simulink model "IEEE123bus_v2019b_Phasor_DPL_ZIPload"  (R2019b)
settings: Solver=VariableStepAuto  StartTime=0.0  StopTime=100  FixedStep=Ts  RelTol=1e-3
InitFcn:
  | a=1; % Loading Factor
  | Ts=0.1;% For Delay Blocks in Voltage Regulator Controls
  | 
  | % Simulation data for the IEEE 123 Node Test Feeder model
  | mi2km = 1.60934;%  miles to km conversion
  | ft2km = 0.0003048; % feet to km conversion
  | ms2F = 1*1e-6/(2*pi*60);% microsiemens to Farads conversion
  | 
  | %% Configuration 1
  | % Series Resitance and Reactance - ohm/mile
  | R_1 = [0.4576 0.1560 0.1535;0.1560 0.4666 0.1580;0.1535 0.1580 0.4615];
  | X_1 = [1.0780 0.5017 0.3849;0.5017 1.0482 0.4236;0.3849 0.4236 1.0651];
  | % charging susceptance - microsiemens/mile
  | B_1 = [5.6765 -1.8319 -0.6982;-1.8319 5.9809 -1.1645;-0.6982 -1.1645 5.3971];
  | 
  | R_1 = R_1/mi2km;
  | L_1 = (X_1/(2*pi*60))/mi2km;
  | C_1 =(B_1*ms2F)/mi2km;
  | 
  | %% Configuration 2 - series reactance - ohm/mile
  | R_2 = [0.4666 0.1580 0.1560;0.1580 0.4615 0.1535;0.1560 0.1535 0.4576];
  | X_2 = [1.0482 0.4236 0.5017;0.4236 1.0651 0.3849;0.5017 0.3849 1.0780];
  | % charging susceptance - microsiemens/mile
  | B_2 = [5.9809 -1.1645 -1.8319;-1.1645 5.3971 -0.6982;-1.8319 -0.6982 5.6765];
  | 
  | R_2 = R_2/mi2km;
  | L_2 = (X_2/(2*pi*60))/mi2km;
  | C_2 =(B_2*ms2F)/mi2km;
  | 
  | %% Configuration 3 - series reactance - ohm/mile
  | R_3 = [0.4615 0.1535 0.1580;0.1535 0.4576 0.1560;0.1580 0.1560 0.4666];
  | X_3 = [1.0651 0.3849 0.4236;0.3849 1.0780 0.5017;0.4236 0.5017 1.0482];
  | % charging susceptance - microsiemens/mile
  | B_3 = [5.3971 -0.6982 -1.1645;-0.6982 5.6765 -1.8319; -1.1645 -1.8319 5.9809];
  | 
  | R_3 = R_3/mi2km;
  | L_3 = (X_3/(2*pi*60))/mi2km;
  | C_3 =(B_3*ms2F)/mi2km;
  | 
  | %% Configuration 4 - series reactance - ohm/mile
  | R_4 = [0.4615 0.1580 0.1535;0.1580 0.4666 0.1560;0.1535 0.1560 0.4576];
  | X_4 = [1.0651 0.4236 0.3849;0.4236 1.0482 0.5017;0.3849 0.5017 1.0780];
  | % charging susceptance - microsiemens/mile
  | B_4 = [5.3971 -1.1645 -0.6982;-1.1645 5.9809 -1.8319;-0.6982 -1.8319 5.6765];
  | 
  | R_4 = R_4/mi2km;
  | L_4 = (X_4/(2*pi*60))/mi2km;
  | C_4 =(B_4*ms2F)/mi2km;
  | 
  | %% Configuration 5 - series reactance - ohm/mile
  | R_5 = [0.4666 0.1560 0.1580;0.1560 0.4576 0.1535;0.1580 0.1535 0.4615];
  | X_5 = [1.0482 0.5017 0.4236;0.5017 1.0780 0.3849;0.4236 0.3849 1.0651];
  | % charging susceptance - microsiemens/mile
  | B_5 = [5.9809 -1.8319 -1.1645;-1.8319 5.6765 -0.6982;-1.1645 -0.6982 5.3971];
  | 
  | R_5 = R_5/mi2km;
  | L_5 = (X_5/(2*pi*60))/mi2km;
  | C_5 =(B_5*ms2F)/mi2km;
  | 
  | %% Configuration 6 - series reactance - ohm/mile
  | ... (+68 lines)
undefined symbols (not defined in the file or in its folder): D1, Delta, find_system, j
libraries: powerlib x886, powerlib_meascontrol x31
(part 4 of 12)

== system IEEE123bus_v2019b_Phasor_DPL_ZIPload/22 Y Z ==
  Controlled Current Source : powerlib/Electrical Sources/Controlled Current Source  Initialize=off  Source_Type=AC  Amplitude=0  Phase=0  Frequency=0  Measurements=None
      settings: SourceProductName=Simscape Electrical
  Embedded MATLAB Function : MATLAB Function  TreatAsAtomicUnit=on
  Gain4 : Gain  Gain=sqrt(2)
  Gain5 : Gain  Gain=1/sqrt(2)
  Memory1 : Memory
  Rc+jXc1 : powerlib/Elements/Series RLC Branch  LConnTagsString=__new0  RConnTagsString=__new0  BranchType=R  Resistance=1e6  Inductance=1.6 / (120*pi) * 2  SetiL0=off  InitialCurrent=0  Capacitance=1e-6  Setx0=off  InitialVoltage=0  Measurements=None
      settings: SourceProductName=Simscape Electrical
  Voltage Measurement1 : powerlib/Measurements/Voltage Measurement  PhasorSimulation=on  OutputType=Complex  PSBequivalent=0
      settings: SourceProductName=Simscape Electrical
  " 2" : PMIOPort  Tag=PMCPort  Side=Left
  " 3" : PMIOPort  Tag=PMCPort  Port=2  Side=Right
  wires:
  Gain4/1 -> Memory1/1
  [v] -> Gain5/1
  Voltage Measurement1/1 -> [v]
  Gain5/1 -> Embedded MATLAB Function/1(Vmeas)
  Memory1/1 -> Controlled Current Source/1
  Embedded MATLAB Function/1(Iinj) -> Gain4/1
  connections:
  Controlled Current Source/LConn1 -- Voltage Measurement1/LConn1 -- " 2"/RConn1 -- Rc+jXc1/LConn1
  " 3"/RConn1 -- Voltage Measurement1/LConn2 -- Rc+jXc1/RConn1 -- Controlled Current Source/RConn1

== system IEEE123bus_v2019b_Phasor_DPL_ZIPload/24 ==
  2 : powerlib/Measurements/Three-Phase V-I Measurement  VoltageMeasurement=phase-to-ground  SetLabelV=on  LabelV=V24  Vpu=off  VpuLL=off  CurrentMeasurement=no  SetLabelI=on  LabelI=I800  Ipu=off  Pbase=100e6  Vbase=24900  OutputType=Complex  PhasorSimulation=on  PSBequivalent=0
      settings: SourceProductName=Simscape Electrical
  Ground82 : powerlib/Elements/Ground  LConnTagsString=a
      settings: SourceProductName=Simscape Electrical
  Ground83 : powerlib/Elements/Ground  LConnTagsString=a
      settings: SourceProductName=Simscape Electrical
  c : PMIOPort  Side=Right
  C : PMIOPort  Port=2  Side=Left
  connections:
  C/RConn1 -- 2/LConn3
  c/RConn1 -- 2/RConn3
  Ground82/LConn1 -- 2/RConn2 -- 2/RConn1
  Ground83/LConn1 -- 2/LConn2 -- 2/LConn1

== system IEEE123bus_v2019b_Phasor_DPL_ZIPload/24 Y PQ ==
  Controlled Current Source : powerlib/Electrical Sources/Controlled Current Source  Initialize=off  Source_Type=AC  Amplitude=0  Phase=0  Frequency=0  Measurements=None
      settings: SourceProductName=Simscape Electrical
  Embedded MATLAB Function : MATLAB Function  TreatAsAtomicUnit=on
  Gain4 : Gain  Gain=sqrt(2)
  Gain5 : Gain  Gain=1/sqrt(2)
  Memory1 : Memory
  Rc+jXc1 : powerlib/Elements/Series RLC Branch  LConnTagsString=__new0  RConnTagsString=__new0  BranchType=R  Resistance=1e6  Inductance=1.6 / (120*pi) * 2  SetiL0=off  InitialCurrent=0  Capacitance=1e-6  Setx0=off  InitialVoltage=0  Measurements=None
      settings: SourceProductName=Simscape Electrical
  Voltage Measurement1 : powerlib/Measurements/Voltage Measurement  PhasorSimulation=on  OutputType=Complex  PSBequivalent=0
      settings: SourceProductName=Simscape Electrical
  " 2" : PMIOPort  Tag=PMCPort  Side=Left
  " 3" : PMIOPort  Tag=PMCPort  Port=2  Side=Right
  wires:
  Embedded MATLAB Function/1(Iinj) -> Gain4/1
  Memory1/1 -> Controlled Current Source/1
  Gain5/1 -> Embedded MATLAB Function/1(Vmeas)
  Voltage Measurement1/1 -> [v]
  [v] -> Gain5/1
  Gain4/1 -> Memory1/1
  connections:
  Controlled Current Source/RConn1 -- Rc+jXc1/RConn1 -- Voltage Measurement1/LConn2 -- " 3"/RConn1
  Rc+jXc1/LConn1 -- " 2"/RConn1 -- Voltage Measurement1/LConn1 -- Controlled Current Source/LConn1

== system IEEE123bus_v2019b_Phasor_DPL_ZIPload/26 ==
  1 : powerlib/Measurements/Three-Phase V-I Measurement  VoltageMeasurement=phase-to-ground  SetLabelV=on  LabelV=V26  Vpu=off  VpuLL=off  CurrentMeasurement=no  SetLabelI=on  LabelI=I800  Ipu=off  Pbase=100e6  Vbase=24900  OutputType=Complex  PhasorSimulation=on  PSBequivalent=0
      settings: SourceProductName=Simscape Electrical
  Ground1 : powerlib/Elements/Ground  LConnTagsString=a
      settings: SourceProductName=Simscape Electrical
  Ground2 : powerlib/Elements/Ground  LConnTagsString=a
      settings: SourceProductName=Simscape Electrical
  A : PMIOPort  Side=Left
  a : PMIOPort  Port=2  Side=Right
  C : PMIOPort  Port=3  Side=Left
  c : PMIOPort  Port=4  Side=Right
  connections:
  1/LConn2 -- Ground2/LConn1
  c/RConn1 -- 1/RConn3
  1/RConn2 -- Ground1/LConn1
  C/RConn1 -- 1/LConn3
  a/RConn1 -- 1/RConn1
  A/RConn1 -- 1/LConn1

== system IEEE123bus_v2019b_Phasor_DPL_ZIPload/27 ==
  1 : powerlib/Measurements/Three-Phase V-I Measurement  VoltageMeasurement=phase-to-ground  SetLabelV=on  LabelV=V27  Vpu=off  VpuLL=off  CurrentMeasurement=no  SetLabelI=on  LabelI=I800  Ipu=off  Pbase=100e6  Vbase=24900  OutputType=Complex  PhasorSimulation=on  PSBequivalent=0
      settings: SourceProductName=Simscape Electrical
  Ground1 : powerlib/Elements/Ground  LConnTagsString=a
      settings: SourceProductName=Simscape Electrical
  Ground2 : powerlib/Elements/Ground  LConnTagsString=a
      settings: SourceProductName=Simscape Electrical
  A : PMIOPort  Side=Left
  a : PMIOPort  Port=2  Side=Right
  C : PMIOPort  Port=3  Side=Left
  c : PMIOPort  Port=4  Side=Right
  connections:
  A/RConn1 -- 1/LConn1
  a/RConn1 -- 1/RConn1
  C/RConn1 -- 1/LConn3
  1/RConn2 -- Ground1/LConn1
  c/RConn1 -- 1/RConn3
  1/LConn2 -- Ground2/LConn1

== system IEEE123bus_v2019b_Phasor_DPL_ZIPload/28 Y I ==
  Controlled Current Source : powerlib/Electrical Sources/Controlled Current Source  Initialize=off  Source_Type=AC  Amplitude=0  Phase=0  Frequency=0  Measurements=None
      settings: SourceProductName=Simscape Electrical
  Embedded MATLAB Function : MATLAB Function  TreatAsAtomicUnit=on
  Gain4 : Gain  Gain=sqrt(2)
  Gain5 : Gain  Gain=1/sqrt(2)
  Memory1 : Memory
  Rc+jXc1 : powerlib/Elements/Series RLC Branch  LConnTagsString=__new0  RConnTagsString=__new0  BranchType=R  Resistance=1e6  Inductance=1.6 / (120*pi) * 2  SetiL0=off  InitialCurrent=0  Capacitance=1e-6  Setx0=off  InitialVoltage=0  Measurements=None
      settings: SourceProductName=Simscape Electrical
  Voltage Measurement1 : powerlib/Measurements/Voltage Measurement  PhasorSimulation=on  OutputType=Complex  PSBequivalent=0
      settings: SourceProductName=Simscape Electrical
  " 2" : PMIOPort  Tag=PMCPort  Side=Left
  " 3" : PMIOPort  Tag=PMCPort  Port=2  Side=Right
  wires:
  Embedded MATLAB Function/1(Iinj) -> Gain4/1
  Memory1/1 -> Controlled Current Source/1
  Gain5/1 -> Embedded MATLAB Function/1(Vmeas)
  Voltage Measurement1/1 -> [v]
  [v] -> Gain5/1
  Gain4/1 -> Memory1/1
  connections:
  Controlled Current Source/RConn1 -- Rc+jXc1/RConn1 -- Voltage Measurement1/LConn2 -- " 3"/RConn1
  Rc+jXc1/LConn1 -- " 2"/RConn1 -- Voltage Measurement1/LConn1 -- Controlled Current Source/LConn1

== system IEEE123bus_v2019b_Phasor_DPL_ZIPload/29 Y Z ==
  Controlled Current Source : powerlib/Electrical Sources/Controlled Current Source  Initialize=off  Source_Type=AC  Amplitude=0  Phase=0  Frequency=0  Measurements=None
      settings: SourceProductName=Simscape Electrical
  Embedded MATLAB Function : MATLAB Function  TreatAsAtomicUnit=on
  Gain4 : Gain  Gain=sqrt(2)
  Gain5 : Gain  Gain=1/sqrt(2)
  Memory1 : Memory
  Rc+jXc1 : powerlib/Elements/Series RLC Branch  LConnTagsString=__new0  RConnTagsString=__new0  BranchType=R  Resistance=1e6  Inductance=1.6 / (120*pi) * 2  SetiL0=off  InitialCurrent=0  Capacitance=1e-6  Setx0=off  InitialVoltage=0  Measurements=None
      settings: SourceProductName=Simscape Electrical
  Voltage Measurement1 : powerlib/Measurements/Voltage Measurement  PhasorSimulation=on  OutputType=Complex  PSBequivalent=0
      settings: SourceProductName=Simscape Electrical
  " 2" : PMIOPort  Tag=PMCPort  Side=Left
  " 3" : PMIOPort  Tag=PMCPort  Port=2  Side=Right
  wires:
  Embedded MATLAB Function/1(Iinj) -> Gain4/1
  Memory1/1 -> Controlled Current Source/1
  Gain5/1 -> Embedded MATLAB Function/1(Vmeas)
  Voltage Measurement1/1 -> [v]
  [v] -> Gain5/1
  Gain4/1 -> Memory1/1
  connections:
  Controlled Current Source/RConn1 -- Rc+jXc1/RConn1 -- Voltage Measurement1/LConn2 -- " 3"/RConn1
  Rc+jXc1/LConn1 -- " 2"/RConn1 -- Voltage Measurement1/LConn1 -- Controlled Current Source/LConn1

== system IEEE123bus_v2019b_Phasor_DPL_ZIPload/3 ==
  2 : powerlib/Measurements/Three-Phase V-I Measurement  VoltageMeasurement=phase-to-ground  SetLabelV=on  LabelV=V3  Vpu=off  VpuLL=off  CurrentMeasurement=no  SetLabelI=on  LabelI=I800  Ipu=off  Pbase=100e6  Vbase=24900  OutputType=Complex  PhasorSimulation=on  PSBequivalent=0
      settings: SourceProductName=Simscape Electrical
  Ground82 : powerlib/Elements/Ground  LConnTagsString=a
      settings: SourceProductName=Simscape Electrical
  Ground83 : powerlib/Elements/Ground  LConnTagsString=a
      settings: SourceProductName=Simscape Electrical
  c : PMIOPort  Side=Right
  C : PMIOPort  Port=2  Side=Left
  connections:
  C/RConn1 -- 2/LConn3
  c/RConn1 -- 2/RConn3
  2/RConn2 -- 2/RConn1 -- Ground82/LConn1
  2/LConn2 -- 2/LConn1 -- Ground83/LConn1

== system IEEE123bus_v2019b_Phasor_DPL_ZIPload/30 Y PQ ==
  Controlled Current Source : powerlib/Electrical Sources/Controlled Current Source  Initialize=off  Source_Type=AC  Amplitude=0  Phase=0  Frequency=0  Measurements=None
      settings: SourceProductName=Simscape Electrical
  Embedded MATLAB Function : MATLAB Function  TreatAsAtomicUnit=on
  Gain4 : Gain  Gain=sqrt(2)
  Gain5 : Gain  Gain=1/sqrt(2)
  Memory1 : Memory
  Rc+jXc1 : powerlib/Elements/Series RLC Branch  LConnTagsString=__new0  RConnTagsString=__new0  BranchType=R  Resistance=1e6  Inductance=1.6 / (120*pi) * 2  SetiL0=off  InitialCurrent=0  Capacitance=1e-6  Setx0=off  InitialVoltage=0  Measurements=None
      settings: SourceProductName=Simscape Electrical
  Voltage Measurement1 : powerlib/Measurements/Voltage Measurement  PhasorSimulation=on  OutputType=Complex  PSBequivalent=0
      settings: SourceProductName=Simscape Electrical
  " 2" : PMIOPort  Tag=PMCPort  Side=Left
  " 3" : PMIOPort  Tag=PMCPort  Port=2  Side=Right
  wires:
  Embedded MATLAB Function/1(Iinj) -> Gain4/1
  Memory1/1 -> Controlled Current Source/1
  Gain5/1 -> Embedded MATLAB Function/1(Vmeas)
  Voltage Measurement1/1 -> [v]
  [v] -> Gain5/1
  Gain4/1 -> Memory1/1
  connections:
  Controlled Current Source/RConn1 -- Rc+jXc1/RConn1 -- Voltage Measurement1/LConn2 -- " 3"/RConn1
  Rc+jXc1/LConn1 -- " 2"/RConn1 -- Voltage Measurement1/LConn1 -- Controlled Current Source/LConn1

== system IEEE123bus_v2019b_Phasor_DPL_ZIPload/31 ==
  2 : powerlib/Measurements/Three-Phase V-I Measurement  VoltageMeasurement=phase-to-ground  SetLabelV=on  LabelV=V31  Vpu=off  VpuLL=off  CurrentMeasurement=no  SetLabelI=on  LabelI=I800  Ipu=off  Pbase=100e6  Vbase=24900  OutputType=Complex  PhasorSimulation=on  PSBequivalent=0
      settings: SourceProductName=Simscape Electrical
  Ground82 : powerlib/Elements/Ground  LConnTagsString=a
      settings: SourceProductName=Simscape Electrical
  Ground83 : powerlib/Elements/Ground  LConnTagsString=a
      settings: SourceProductName=Simscape Electrical
  c : PMIOPort  Side=Right
  C : PMIOPort  Port=2  Side=Left
  connections:
  2/LConn1 -- 2/LConn2 -- Ground83/LConn1
  2/RConn1 -- 2/RConn2 -- Ground82/LConn1
  c/RConn1 -- 2/RConn3
  C/RConn1 -- 2/LConn3

== system IEEE123bus_v2019b_Phasor_DPL_ZIPload/31 Y PQ ==
  Controlled Current Source : powerlib/Electrical Sources/Controlled Current Source  Initialize=off  Source_Type=AC  Amplitude=0  Phase=0  Frequency=0  Measurements=None
      settings: SourceProductName=Simscape Electrical
  Embedded MATLAB Function : MATLAB Function  TreatAsAtomicUnit=on
  Gain4 : Gain  Gain=sqrt(2)
  Gain5 : Gain  Gain=1/sqrt(2)
  Memory1 : Memory
  Rc+jXc1 : powerlib/Elements/Series RLC Branch  LConnTagsString=__new0  RConnTagsString=__new0  BranchType=R  Resistance=1e6  Inductance=1.6 / (120*pi) * 2  SetiL0=off  InitialCurrent=0  Capacitance=1e-6  Setx0=off  InitialVoltage=0  Measurements=None
      settings: SourceProductName=Simscape Electrical
  Voltage Measurement1 : powerlib/Measurements/Voltage Measurement  PhasorSimulation=on  OutputType=Complex  PSBequivalent=0
      settings: SourceProductName=Simscape Electrical
  " 2" : PMIOPort  Tag=PMCPort  Side=Left
  " 3" : PMIOPort  Tag=PMCPort  Port=2  Side=Right
  wires:
  Gain4/1 -> Memory1/1
  [v] -> Gain5/1
  Voltage Measurement1/1 -> [v]
  Gain5/1 -> Embedded MATLAB Function/1(Vmeas)
  Memory1/1 -> Controlled Current Source/1
  Embedded MATLAB Function/1(Iinj) -> Gain4/1
  connections:
  Controlled Current Source/LConn1 -- Voltage Measurement1/LConn1 -- " 2"/RConn1 -- Rc+jXc1/LConn1
  " 3"/RConn1 -- Voltage Measurement1/LConn2 -- Rc+jXc1/RConn1 -- Controlled Current Source/RConn1

== system IEEE123bus_v2019b_Phasor_DPL_ZIPload/32 ==
  2 : powerlib/Measurements/Three-Phase V-I Measurement  VoltageMeasurement=phase-to-ground  SetLabelV=on  LabelV=V32  Vpu=off  VpuLL=off  CurrentMeasurement=no  SetLabelI=on  LabelI=I800  Ipu=off  Pbase=100e6  Vbase=24900  OutputType=Complex  PhasorSimulation=on  PSBequivalent=0
      settings: SourceProductName=Simscape Electrical
  Ground82 : powerlib/Elements/Ground  LConnTagsString=a
      settings: SourceProductName=Simscape Electrical
  Ground83 : powerlib/Elements/Ground  LConnTagsString=a
      settings: SourceProductName=Simscape Electrical
  c : PMIOPort  Side=Right
  C : PMIOPort  Port=2  Side=Left
  connections:
  C/RConn1 -- 2/LConn3
  c/RConn1 -- 2/RConn3
  Ground82/LConn1 -- 2/RConn2 -- 2/RConn1
  Ground83/LConn1 -- 2/LConn2 -- 2/LConn1

== system IEEE123bus_v2019b_Phasor_DPL_ZIPload/32 Y PQ ==
  Controlled Current Source : powerlib/Electrical Sources/Controlled Current Source  Initialize=off  Source_Type=AC  Amplitude=0  Phase=0  Frequency=0  Measurements=None
      settings: SourceProductName=Simscape Electrical
  Embedded MATLAB Function : MATLAB Function  TreatAsAtomicUnit=on
  Gain4 : Gain  Gain=sqrt(2)
  Gain5 : Gain  Gain=1/sqrt(2)
  Memory1 : Memory
  Rc+jXc1 : powerlib/Elements/Series RLC Branch  LConnTagsString=__new0  RConnTagsString=__new0  BranchType=R  Resistance=1e6  Inductance=1.6 / (120*pi) * 2  SetiL0=off  InitialCurrent=0  Capacitance=1e-6  Setx0=off  InitialVoltage=0  Measurements=None
      settings: SourceProductName=Simscape Electrical
  Voltage Measurement1 : powerlib/Measurements/Voltage Measurement  PhasorSimulation=on  OutputType=Complex  PSBequivalent=0
      settings: SourceProductName=Simscape Electrical
  " 2" : PMIOPort  Tag=PMCPort  Side=Left
  " 3" : PMIOPort  Tag=PMCPort  Port=2  Side=Right
  wires:
  Embedded MATLAB Function/1(Iinj) -> Gain4/1
  Memory1/1 -> Controlled Current Source/1
  Gain5/1 -> Embedded MATLAB Function/1(Vmeas)
  Voltage Measurement1/1 -> [v]
  [v] -> Gain5/1
  Gain4/1 -> Memory1/1
  connections:
  Controlled Current Source/RConn1 -- Rc+jXc1/RConn1 -- Voltage Measurement1/LConn2 -- " 3"/RConn1
  Rc+jXc1/LConn1 -- " 2"/RConn1 -- Voltage Measurement1/LConn1 -- Controlled Current Source/LConn1

== system IEEE123bus_v2019b_Phasor_DPL_ZIPload/33 ==
  2 : powerlib/Measurements/Three-Phase V-I Measurement  VoltageMeasurement=phase-to-ground  SetLabelV=on  LabelV=V33  Vpu=off  VpuLL=off  CurrentMeasurement=no  SetLabelI=on  LabelI=I800  Ipu=off  Pbase=100e6  Vbase=24900  OutputType=Complex  PhasorSimulation=on  PSBequivalent=0
      settings: SourceProductName=Simscape Electrical
  Ground82 : powerlib/Elements/Ground  LConnTagsString=a
      settings: SourceProductName=Simscape Electrical
  Ground83 : powerlib/Elements/Ground  LConnTagsString=a
      settings: SourceProductName=Simscape Electrical
  a : PMIOPort  Side=Right
  A : PMIOPort  Port=2  Side=Left
  connections:
  A/RConn1 -- 2/LConn1
  a/RConn1 -- 2/RConn1
  Ground83/LConn1 -- 2/LConn2 -- 2/LConn3
  Ground82/LConn1 -- 2/RConn2 -- 2/RConn3

== system IEEE123bus_v2019b_Phasor_DPL_ZIPload/33 Y I ==
  Controlled Current Source : powerlib/Electrical Sources/Controlled Current Source  Initialize=off  Source_Type=AC  Amplitude=0  Phase=0  Frequency=0  Measurements=None
      settings: SourceProductName=Simscape Electrical
  Embedded MATLAB Function : MATLAB Function  TreatAsAtomicUnit=on
  Gain4 : Gain  Gain=sqrt(2)
  Gain5 : Gain  Gain=1/sqrt(2)
  Memory1 : Memory
  Rc+jXc1 : powerlib/Elements/Series RLC Branch  LConnTagsString=__new0  RConnTagsString=__new0  BranchType=R  Resistance=1e6  Inductance=1.6 / (120*pi) * 2  SetiL0=off  InitialCurrent=0  Capacitance=1e-6  Setx0=off  InitialVoltage=0  Measurements=None
      settings: SourceProductName=Simscape Electrical
  Voltage Measurement1 : powerlib/Measurements/Voltage Measurement  PhasorSimulation=on  OutputType=Complex  PSBequivalent=0
      settings: SourceProductName=Simscape Electrical
  " 2" : PMIOPort  Tag=PMCPort  Side=Left
  " 3" : PMIOPort  Tag=PMCPort  Port=2  Side=Right
  wires:
  Embedded MATLAB Function/1(Iinj) -> Gain4/1
  Memory1/1 -> Controlled Current Source/1
  Gain5/1 -> Embedded MATLAB Function/1(Vmeas)
  Voltage Measurement1/1 -> [v]
  [v] -> Gain5/1
  Gain4/1 -> Memory1/1
  connections:
  Controlled Current Source/RConn1 -- Rc+jXc1/RConn1 -- Voltage Measurement1/LConn2 -- " 3"/RConn1
  Rc+jXc1/LConn1 -- " 2"/RConn1 -- Voltage Measurement1/LConn1 -- Controlled Current Source/LConn1

== system IEEE123bus_v2019b_Phasor_DPL_ZIPload/34 ==
  2 : powerlib/Measurements/Three-Phase V-I Measurement  VoltageMeasurement=phase-to-ground  SetLabelV=on  LabelV=V34  Vpu=off  VpuLL=off  CurrentMeasurement=no  SetLabelI=on  LabelI=I800  Ipu=off  Pbase=100e6  Vbase=24900  OutputType=Complex  PhasorSimulation=on  PSBequivalent=0
      settings: SourceProductName=Simscape Electrical
  Ground82 : powerlib/Elements/Ground  LConnTagsString=a
      settings: SourceProductName=Simscape Electrical
  Ground83 : powerlib/Elements/Ground  LConnTagsString=a
      settings: SourceProductName=Simscape Electrical
  c : PMIOPort  Side=Right
  C : PMIOPort  Port=2  Side=Left
  connections:
  C/RConn1 -- 2/LConn3
  c/RConn1 -- 2/RConn3
  2/RConn2 -- 2/RConn1 -- Ground82/LConn1
  2/LConn2 -- 2/LConn1 -- Ground83/LConn1

== system IEEE123bus_v2019b_Phasor_DPL_ZIPload/34 Y Z ==
  Controlled Current Source : powerlib/Electrical Sources/Controlled Current Source  Initialize=off  Source_Type=AC  Amplitude=0  Phase=0  Frequency=0  Measurements=None
      settings: SourceProductName=Simscape Electrical
  Embedded MATLAB Function : MATLAB Function  TreatAsAtomicUnit=on
  Gain4 : Gain  Gain=sqrt(2)
  Gain5 : Gain  Gain=1/sqrt(2)
  Memory1 : Memory
  Rc+jXc1 : powerlib/Elements/Series RLC Branch  LConnTagsString=__new0  RConnTagsString=__new0  BranchType=R  Resistance=1e6  Inductance=1.6 / (120*pi) * 2  SetiL0=off  InitialCurrent=0  Capacitance=1e-6  Setx0=off  InitialVoltage=0  Measurements=None
      settings: SourceProductName=Simscape Electrical
  Voltage Measurement1 : powerlib/Measurements/Voltage Measurement  PhasorSimulation=on  OutputType=Complex  PSBequivalent=0
      settings: SourceProductName=Simscape Electrical
  " 2" : PMIOPort  Tag=PMCPort  Side=Left
  " 3" : PMIOPort  Tag=PMCPort  Port=2  Side=Right
  wires:
  Embedded MATLAB Function/1(Iinj) -> Gain4/1
  Memory1/1 -> Controlled Current Source/1
  Gain5/1 -> Embedded MATLAB Function/1(Vmeas)
  Voltage Measurement1/1 -> [v]
  [v] -> Gain5/1
  Gain4/1 -> Memory1/1
  connections:
  Controlled Current Source/RConn1 -- Rc+jXc1/RConn1 -- Voltage Measurement1/LConn2 -- " 3"/RConn1
  Rc+jXc1/LConn1 -- " 2"/RConn1 -- Voltage Measurement1/LConn1 -- Controlled Current Source/LConn1

== system IEEE123bus_v2019b_Phasor_DPL_ZIPload/35 D PQ ==
  Controlled Current Source : powerlib/Electrical Sources/Controlled Current Source  Initialize=off  Source_Type=AC  Amplitude=0  Phase=0  Frequency=0  Measurements=None
      settings: SourceProductName=Simscape Electrical
  Embedded MATLAB Function : MATLAB Function  TreatAsAtomicUnit=on
  Gain4 : Gain  Gain=sqrt(2)
  Gain5 : Gain  Gain=1/sqrt(2)
  Memory1 : Memory
  Rc+jXc1 : powerlib/Elements/Series RLC Branch  LConnTagsString=__new0  RConnTagsString=__new0  BranchType=R  Resistance=1e6  Inductance=1.6 / (120*pi) * 2  SetiL0=off  InitialCurrent=0  Capacitance=1e-6  Setx0=off  InitialVoltage=0  Measurements=None
      settings: SourceProductName=Simscape Electrical
  Voltage Measurement1 : powerlib/Measurements/Voltage Measurement  PhasorSimulation=on  OutputType=Complex  PSBequivalent=0
      settings: SourceProductName=Simscape Electrical
  " 2" : PMIOPort  Tag=PMCPort  Side=Left
  " 3" : PMIOPort  Tag=PMCPort  Port=2  Side=Right
  wires:
  Embedded MATLAB Function/1(Iinj) -> Gain4/1
  Memory1/1 -> Controlled Current Source/1
  Gain5/1 -> Embedded MATLAB Function/1(Vmeas)
  Voltage Measurement1/1 -> [v]
  [v] -> Gain5/1
  Gain4/1 -> Memory1/1
  connections:
  Controlled Current Source/RConn1 -- Rc+jXc1/RConn1 -- Voltage Measurement1/LConn2 -- " 3"/RConn1
  Rc+jXc1/LConn1 -- " 2"/RConn1 -- Voltage Measurement1/LConn1 -- Controlled Current Source/LConn1

== system IEEE123bus_v2019b_Phasor_DPL_ZIPload/36 ==
  1 : powerlib/Measurements/Three-Phase V-I Measurement  VoltageMeasurement=phase-to-ground  SetLabelV=on  LabelV=V36  Vpu=off  VpuLL=off  CurrentMeasurement=no  SetLabelI=on  LabelI=I800  Ipu=off  Pbase=100e6  Vbase=24900  OutputType=Complex  PhasorSimulation=on  PSBequivalent=0
      settings: SourceProductName=Simscape Electrical
  Ground1 : powerlib/Elements/Ground  LConnTagsString=a
      settings: SourceProductName=Simscape Electrical
  Ground2 : powerlib/Elements/Ground  LConnTagsString=a
      settings: SourceProductName=Simscape Electrical
  A : PMIOPort  Side=Left
  a : PMIOPort  Port=2  Side=Right
  B : PMIOPort  Port=3  Side=Left
  b : PMIOPort  Port=4  Side=Right
  connections:
  A/RConn1 -- 1/LConn1
  a/RConn1 -- 1/RConn1
  b/RConn1 -- 1/RConn2
  1/RConn3 -- Ground1/LConn1
  B/RConn1 -- 1/LConn2
  1/LConn3 -- Ground2/LConn1

== system IEEE123bus_v2019b_Phasor_DPL_ZIPload/37 ==
  2 : powerlib/Measurements/Three-Phase V-I Measurement  VoltageMeasurement=phase-to-ground  SetLabelV=on  LabelV=V37  Vpu=off  VpuLL=off  CurrentMeasurement=no  SetLabelI=on  LabelI=I800  Ipu=off  Pbase=100e6  Vbase=24900  OutputType=Complex  PhasorSimulation=on  PSBequivalent=0
      settings: SourceProductName=Simscape Electrical
  Ground82 : powerlib/Elements/Ground  LConnTagsString=a
      settings: SourceProductName=Simscape Electrical
  Ground83 : powerlib/Elements/Ground  LConnTagsString=a
      settings: SourceProductName=Simscape Electrical
  a : PMIOPort  Side=Right
  A : PMIOPort  Port=2  Side=Left
  connections:
  2/RConn3 -- 2/RConn2 -- Ground82/LConn1
  2/LConn3 -- 2/LConn2 -- Ground83/LConn1
  a/RConn1 -- 2/RConn1
  A/RConn1 -- 2/LConn1

== system IEEE123bus_v2019b_Phasor_DPL_ZIPload/37 Y Z ==
  Controlled Current Source : powerlib/Electrical Sources/Controlled Current Source  Initialize=off  Source_Type=AC  Amplitude=0  Phase=0  Frequency=0  Measurements=None
      settings: SourceProductName=Simscape Electrical
  Embedded MATLAB Function : MATLAB Function  TreatAsAtomicUnit=on
  Gain4 : Gain  Gain=sqrt(2)
  Gain5 : Gain  Gain=1/sqrt(2)
  Memory1 : Memory
  Rc+jXc1 : powerlib/Elements/Series RLC Branch  LConnTagsString=__new0  RConnTagsString=__new0  BranchType=R  Resistance=1e6  Inductance=1.6 / (120*pi) * 2  SetiL0=off  InitialCurrent=0  Capacitance=1e-6  Setx0=off  InitialVoltage=0  Measurements=None
      settings: SourceProductName=Simscape Electrical
  Voltage Measurement1 : powerlib/Measurements/Voltage Measurement  PhasorSimulation=on  OutputType=Complex  PSBequivalent=0
      settings: SourceProductName=Simscape Electrical
  " 2" : PMIOPort  Tag=PMCPort  Side=Left
  " 3" : PMIOPort  Tag=PMCPort  Port=2  Side=Right
  wires:
  Embedded MATLAB Function/1(Iinj) -> Gain4/1
  Memory1/1 -> Controlled Current Source/1
  Gain5/1 -> Embedded MATLAB Function/1(Vmeas)
  Voltage Measurement1/1 -> [v]
  [v] -> Gain5/1
  Gain4/1 -> Memory1/1
  connections:
  Controlled Current Source/RConn1 -- Rc+jXc1/RConn1 -- Voltage Measurement1/LConn2 -- " 3"/RConn1
  Rc+jXc1/LConn1 -- " 2"/RConn1 -- Voltage Measurement1/LConn1 -- Controlled Current Source/LConn1

== system IEEE123bus_v2019b_Phasor_DPL_ZIPload/38 ==
  2 : powerlib/Measurements/Three-Phase V-I Measurement  VoltageMeasurement=phase-to-ground  SetLabelV=on  LabelV=V38  Vpu=off  VpuLL=off  CurrentMeasurement=no  SetLabelI=on  LabelI=I800  Ipu=off  Pbase=100e6  Vbase=24900  OutputType=Complex  PhasorSimulation=on  PSBequivalent=0
      settings: SourceProductName=Simscape Electrical
  Ground82 : powerlib/Elements/Ground  LConnTagsString=a
      settings: SourceProductName=Simscape Electrical
  Ground83 : powerlib/Elements/Ground  LConnTagsString=a
      settings: SourceProductName=Simscape Electrical
  b : PMIOPort  Side=Right
  B : PMIOPort  Port=2  Side=Left
  connections:
  Ground82/LConn1 -- 2/RConn3 -- 2/RConn1
  Ground83/LConn1 -- 2/LConn3 -- 2/LConn1
  2/RConn2 -- b/RConn1
  2/LConn2 -- B/RConn1

== system IEEE123bus_v2019b_Phasor_DPL_ZIPload/38 Y I ==
  Controlled Current Source : powerlib/Electrical Sources/Controlled Current Source  Initialize=off  Source_Type=AC  Amplitude=0  Phase=0  Frequency=0  Measurements=None
      settings: SourceProductName=Simscape Electrical
  Embedded MATLAB Function : MATLAB Function  TreatAsAtomicUnit=on
  Gain4 : Gain  Gain=sqrt(2)
  Gain5 : Gain  Gain=1/sqrt(2)
  Memory1 : Memory
  Rc+jXc1 : powerlib/Elements/Series RLC Branch  LConnTagsString=__new0  RConnTagsString=__new0  BranchType=R  Resistance=1e6  Inductance=1.6 / (120*pi) * 2  SetiL0=off  InitialCurrent=0  Capacitance=1e-6  Setx0=off  InitialVoltage=0  Measurements=None
      settings: SourceProductName=Simscape Electrical
  Voltage Measurement1 : powerlib/Measurements/Voltage Measurement  PhasorSimulation=on  OutputType=Complex  PSBequivalent=0
      settings: SourceProductName=Simscape Electrical
  " 2" : PMIOPort  Tag=PMCPort  Side=Left
  " 3" : PMIOPort  Tag=PMCPort  Port=2  Side=Right
  wires:
  Gain4/1 -> Memory1/1
  [v] -> Gain5/1
  Voltage Measurement1/1 -> [v]
  Gain5/1 -> Embedded MATLAB Function/1(Vmeas)
  Memory1/1 -> Controlled Current Source/1
  Embedded MATLAB Function/1(Iinj) -> Gain4/1
  connections:
  Controlled Current Source/LConn1 -- Voltage Measurement1/LConn1 -- " 2"/RConn1 -- Rc+jXc1/LConn1
  " 3"/RConn1 -- Voltage Measurement1/LConn2 -- Rc+jXc1/RConn1 -- Controlled Current Source/RConn1

== system IEEE123bus_v2019b_Phasor_DPL_ZIPload/39 ==
  2 : powerlib/Measurements/Three-Phase V-I Measurement  VoltageMeasurement=phase-to-ground  SetLabelV=on  LabelV=V39  Vpu=off  VpuLL=off  CurrentMeasurement=no  SetLabelI=on  LabelI=I800  Ipu=off  Pbase=100e6  Vbase=24900  OutputType=Complex  PhasorSimulation=on  PSBequivalent=0
      settings: SourceProductName=Simscape Electrical
  Ground82 : powerlib/Elements/Ground  LConnTagsString=a
      settings: SourceProductName=Simscape Electrical
  Ground83 : powerlib/Elements/Ground  LConnTagsString=a
      settings: SourceProductName=Simscape Electrical
  b : PMIOPort  Side=Right
  B : PMIOPort  Port=2  Side=Left
  connections:
  2/LConn2 -- B/RConn1
  2/RConn2 -- b/RConn1
  2/LConn1 -- 2/LConn3 -- Ground83/LConn1
  2/RConn1 -- 2/RConn3 -- Ground82/LConn1

== system IEEE123bus_v2019b_Phasor_DPL_ZIPload/39 Y PQ ==
  Controlled Current Source : powerlib/Electrical Sources/Controlled Current Source  Initialize=off  Source_Type=AC  Amplitude=0  Phase=0  Frequency=0  Measurements=None
      settings: SourceProductName=Simscape Electrical
  Embedded MATLAB Function : MATLAB Function  TreatAsAtomicUnit=on
  Gain4 : Gain  Gain=sqrt(2)
  Gain5 : Gain  Gain=1/sqrt(2)
  Memory1 : Memory
  Rc+jXc1 : powerlib/Elements/Series RLC Branch  LConnTagsString=__new0  RConnTagsString=__new0  BranchType=R  Resistance=1e6  Inductance=1.6 / (120*pi) * 2  SetiL0=off  InitialCurrent=0  Capacitance=1e-6  Setx0=off  InitialVoltage=0  Measurements=None
      settings: SourceProductName=Simscape Electrical
  Voltage Measurement1 : powerlib/Measurements/Voltage Measurement  PhasorSimulation=on  OutputType=Complex  PSBequivalent=0
      settings: SourceProductName=Simscape Electrical
  " 2" : PMIOPort  Tag=PMCPort  Side=Left
  " 3" : PMIOPort  Tag=PMCPort  Port=2  Side=Right
  wires:
  Gain4/1 -> Memory1/1
  [v] -> Gain5/1
  Voltage Measurement1/1 -> [v]
  Gain5/1 -> Embedded MATLAB Function/1(Vmeas)
  Memory1/1 -> Controlled Current Source/1
  Embedded MATLAB Function/1(Iinj) -> Gain4/1
  connections:
  Controlled Current Source/LConn1 -- Voltage Measurement1/LConn1 -- " 2"/RConn1 -- Rc+jXc1/LConn1
  " 3"/RConn1 -- Voltage Measurement1/LConn2 -- Rc+jXc1/RConn1 -- Controlled Current Source/RConn1

== system IEEE123bus_v2019b_Phasor_DPL_ZIPload/4 ==
  2 : powerlib/Measurements/Three-Phase V-I Measurement  VoltageMeasurement=phase-to-ground  SetLabelV=on  LabelV=V4  Vpu=off  VpuLL=off  CurrentMeasurement=no  SetLabelI=on  LabelI=I4  Ipu=off  Pbase=100e6  Vbase=24900  OutputType=Complex  PhasorSimulation=on  PSBequivalent=0
      settings: SourceProductName=Simscape Electrical
  Ground82 : powerlib/Elements/Ground  LConnTagsString=a
      settings: SourceProductName=Simscape Electrical
  Ground83 : powerlib/Elements/Ground  LConnTagsString=a
      settings: SourceProductName=Simscape Electrical
  c : PMIOPort  Side=Right
  C : PMIOPort  Port=2  Side=Left
  connections:
  Ground83/LConn1 -- 2/LConn1 -- 2/LConn2
  Ground82/LConn1 -- 2/RConn1 -- 2/RConn2
  c/RConn1 -- 2/RConn3
  C/RConn1 -- 2/LConn3

== system IEEE123bus_v2019b_Phasor_DPL_ZIPload/41 ==
  2 : powerlib/Measurements/Three-Phase V-I Measurement  VoltageMeasurement=phase-to-ground  SetLabelV=on  LabelV=V41  Vpu=off  VpuLL=off  CurrentMeasurement=no  SetLabelI=on  LabelI=I800  Ipu=off  Pbase=100e6  Vbase=24900  OutputType=Complex  PhasorSimulation=on  PSBequivalent=0
      settings: SourceProductName=Simscape Electrical
  Ground82 : powerlib/Elements/Ground  LConnTagsString=a
      settings: SourceProductName=Simscape Electrical
  Ground83 : powerlib/Elements/Ground  LConnTagsString=a
      settings: SourceProductName=Simscape Electrical
  c : PMIOPort  Side=Right
  C : PMIOPort  Port=2  Side=Left
  connections:
  2/LConn1 -- 2/LConn2 -- Ground83/LConn1
  2/RConn1 -- 2/RConn2 -- Ground82/LConn1
  c/RConn1 -- 2/RConn3
  C/RConn1 -- 2/LConn3

== system IEEE123bus_v2019b_Phasor_DPL_ZIPload/41 Y PQ ==
  Controlled Current Source : powerlib/Electrical Sources/Controlled Current Source  Initialize=off  Source_Type=AC  Amplitude=0  Phase=0  Frequency=0  Measurements=None
      settings: SourceProductName=Simscape Electrical
  Embedded MATLAB Function : MATLAB Function  TreatAsAtomicUnit=on
  Gain4 : Gain  Gain=sqrt(2)
  Gain5 : Gain  Gain=1/sqrt(2)
  Memory1 : Memory
  Rc+jXc1 : powerlib/Elements/Series RLC Branch  LConnTagsString=__new0  RConnTagsString=__new0  BranchType=R  Resistance=1e6  Inductance=1.6 / (120*pi) * 2  SetiL0=off  InitialCurrent=0  Capacitance=1e-6  Setx0=off  InitialVoltage=0  Measurements=None
      settings: SourceProductName=Simscape Electrical
  Voltage Measurement1 : powerlib/Measurements/Voltage Measurement  PhasorSimulation=on  OutputType=Complex  PSBequivalent=0
      settings: SourceProductName=Simscape Electrical
  " 2" : PMIOPort  Tag=PMCPort  Side=Left
  " 3" : PMIOPort  Tag=PMCPort  Port=2  Side=Right
  wires:
  Gain4/1 -> Memory1/1
  [v] -> Gain5/1
  Voltage Measurement1/1 -> [v]
  Gain5/1 -> Embedded MATLAB Function/1(Vmeas)
  Memory1/1 -> Controlled Current Source/1
  Embedded MATLAB Function/1(Iinj) -> Gain4/1
  connections:
  Controlled Current Source/LConn1 -- Voltage Measurement1/LConn1 -- " 2"/RConn1 -- Rc+jXc1/LConn1
  " 3"/RConn1 -- Voltage Measurement1/LConn2 -- Rc+jXc1/RConn1 -- Controlled Current Source/RConn1

== system IEEE123bus_v2019b_Phasor_DPL_ZIPload/42 Y PQ ==
  Controlled Current Source : powerlib/Electrical Sources/Controlled Current Source  Initialize=off  Source_Type=AC  Amplitude=0  Phase=0  Frequency=0  Measurements=None
      settings: SourceProductName=Simscape Electrical
  Embedded MATLAB Function : MATLAB Function  TreatAsAtomicUnit=on
  Gain4 : Gain  Gain=sqrt(2)
  Gain5 : Gain  Gain=1/sqrt(2)
  Memory1 : Memory
  Rc+jXc1 : powerlib/Elements/Series RLC Branch  LConnTagsString=__new0  RConnTagsString=__new0  BranchType=R  Resistance=1e6  Inductance=1.6 / (120*pi) * 2  SetiL0=off  InitialCurrent=0  Capacitance=1e-6  Setx0=off  InitialVoltage=0  Measurements=None
      settings: SourceProductName=Simscape Electrical
  Voltage Measurement1 : powerlib/Measurements/Voltage Measurement  PhasorSimulation=on  OutputType=Complex  PSBequivalent=0
      settings: SourceProductName=Simscape Electrical
  " 2" : PMIOPort  Tag=PMCPort  Side=Left
  " 3" : PMIOPort  Tag=PMCPort  Port=2  Side=Right
  wires:
  Embedded MATLAB Function/1(Iinj) -> Gain4/1
  Memory1/1 -> Controlled Current Source/1
  Gain5/1 -> Embedded MATLAB Function/1(Vmeas)
  Voltage Measurement1/1 -> [v]
  [v] -> Gain5/1
  Gain4/1 -> Memory1/1
  connections:
  Controlled Current Source/RConn1 -- Rc+jXc1/RConn1 -- Voltage Measurement1/LConn2 -- " 3"/RConn1
  Rc+jXc1/LConn1 -- " 2"/RConn1 -- Voltage Measurement1/LConn1 -- Controlled Current Source/LConn1

== system IEEE123bus_v2019b_Phasor_DPL_ZIPload/43 ==
  2 : powerlib/Measurements/Three-Phase V-I Measurement  VoltageMeasurement=phase-to-ground  SetLabelV=on  LabelV=V43  Vpu=off  VpuLL=off  CurrentMeasurement=no  SetLabelI=on  LabelI=I800  Ipu=off  Pbase=100e6  Vbase=24900  OutputType=Complex  PhasorSimulation=on  PSBequivalent=0
      settings: SourceProductName=Simscape Electrical
  Ground82 : powerlib/Elements/Ground  LConnTagsString=a
      settings: SourceProductName=Simscape Electrical
  Ground83 : powerlib/Elements/Ground  LConnTagsString=a
      settings: SourceProductName=Simscape Electrical
  b : PMIOPort  Side=Right
  B : PMIOPort  Port=2  Side=Left
  connections:
  2/LConn2 -- B/RConn1
  2/RConn2 -- b/RConn1
  2/LConn1 -- 2/LConn3 -- Ground83/LConn1
  2/RConn1 -- 2/RConn3 -- Ground82/LConn1

== system IEEE123bus_v2019b_Phasor_DPL_ZIPload/43 Y Z ==
  Controlled Current Source : powerlib/Electrical Sources/Controlled Current Source  Initialize=off  Source_Type=AC  Amplitude=0  Phase=0  Frequency=0  Measurements=None
      settings: SourceProductName=Simscape Electrical
  Embedded MATLAB Function : MATLAB Function  TreatAsAtomicUnit=on
  Gain4 : Gain  Gain=sqrt(2)
  Gain5 : Gain  Gain=1/sqrt(2)
  Memory1 : Memory
  Rc+jXc1 : powerlib/Elements/Series RLC Branch  LConnTagsString=__new0  RConnTagsString=__new0  BranchType=R  Resistance=1e6  Inductance=1.6 / (120*pi) * 2  SetiL0=off  InitialCurrent=0  Capacitance=1e-6  Setx0=off  InitialVoltage=0  Measurements=None
      settings: SourceProductName=Simscape Electrical
  Voltage Measurement1 : powerlib/Measurements/Voltage Measurement  PhasorSimulation=on  OutputType=Complex  PSBequivalent=0
      settings: SourceProductName=Simscape Electrical
  " 2" : PMIOPort  Tag=PMCPort  Side=Left
  " 3" : PMIOPort  Tag=PMCPort  Port=2  Side=Right
  wires:
  Embedded MATLAB Function/1(Iinj) -> Gain4/1
  Memory1/1 -> Controlled Current Source/1
  Gain5/1 -> Embedded MATLAB Function/1(Vmeas)
  Voltage Measurement1/1 -> [v]
  [v] -> Gain5/1
  Gain4/1 -> Memory1/1
  connections:
  Controlled Current Source/RConn1 -- Rc+jXc1/RConn1 -- Voltage Measurement1/LConn2 -- " 3"/RConn1
  Rc+jXc1/LConn1 -- " 2"/RConn1 -- Voltage Measurement1/LConn1 -- Controlled Current Source/LConn1

== system IEEE123bus_v2019b_Phasor_DPL_ZIPload/45 ==
  2 : powerlib/Measurements/Three-Phase V-I Measurement  VoltageMeasurement=phase-to-ground  SetLabelV=on  LabelV=V45  Vpu=off  VpuLL=off  CurrentMeasurement=no  SetLabelI=on  LabelI=I800  Ipu=off  Pbase=100e6  Vbase=24900  OutputType=Complex  PhasorSimulation=on  PSBequivalent=0
      settings: SourceProductName=Simscape Electrical
  Ground82 : powerlib/Elements/Ground  LConnTagsString=a
      settings: SourceProductName=Simscape Electrical
  Ground83 : powerlib/Elements/Ground  LConnTagsString=a
      settings: SourceProductName=Simscape Electrical
  a : PMIOPort  Side=Right
  A : PMIOPort  Port=2  Side=Left
  connections:
  2/RConn3 -- 2/RConn2 -- Ground82/LConn1
  2/LConn3 -- 2/LConn2 -- Ground83/LConn1
  a/RConn1 -- 2/RConn1
  A/RConn1 -- 2/LConn1

== system IEEE123bus_v2019b_Phasor_DPL_ZIPload/45 Y I ==
  Controlled Current Source : powerlib/Electrical Sources/Controlled Current Source  Initialize=off  Source_Type=AC  Amplitude=0  Phase=0  Frequency=0  Measurements=None
      settings: SourceProductName=Simscape Electrical
  Embedded MATLAB Function : MATLAB Function  TreatAsAtomicUnit=on
  Gain4 : Gain  Gain=sqrt(2)
  Gain5 : Gain  Gain=1/sqrt(2)
  Memory1 : Memory
  Rc+jXc1 : powerlib/Elements/Series RLC Branch  LConnTagsString=__new0  RConnTagsString=__new0  BranchType=R  Resistance=1e6  Inductance=1.6 / (120*pi) * 2  SetiL0=off  InitialCurrent=0  Capacitance=1e-6  Setx0=off  InitialVoltage=0  Measurements=None
      settings: SourceProductName=Simscape Electrical
  Voltage Measurement1 : powerlib/Measurements/Voltage Measurement  PhasorSimulation=on  OutputType=Complex  PSBequivalent=0
      settings: SourceProductName=Simscape Electrical
  " 2" : PMIOPort  Tag=PMCPort  Side=Left
  " 3" : PMIOPort  Tag=PMCPort  Port=2  Side=Right
  wires:
  Embedded MATLAB Function/1(Iinj) -> Gain4/1
  Memory1/1 -> Controlled Current Source/1
  Gain5/1 -> Embedded MATLAB Function/1(Vmeas)
  Voltage Measurement1/1 -> [v]
  [v] -> Gain5/1
  Gain4/1 -> Memory1/1
  connections:
  Controlled Current Source/RConn1 -- Rc+jXc1/RConn1 -- Voltage Measurement1/LConn2 -- " 3"/RConn1
  Rc+jXc1/LConn1 -- " 2"/RConn1 -- Voltage Measurement1/LConn1 -- Controlled Current Source/LConn1

== system IEEE123bus_v2019b_Phasor_DPL_ZIPload/46 ==
  2 : powerlib/Measurements/Three-Phase V-I Measurement  VoltageMeasurement=phase-to-ground  SetLabelV=on  LabelV=V46  Vpu=off  VpuLL=off  CurrentMeasurement=no  SetLabelI=on  LabelI=I800  Ipu=off  Pbase=100e6  Vbase=24900  OutputType=Complex  PhasorSimulation=on  PSBequivalent=0
      settings: SourceProductName=Simscape Electrical
  Ground82 : powerlib/Elements/Ground  LConnTagsString=a
      settings: SourceProductName=Simscape Electrical
  Ground83 : powerlib/Elements/Ground  LConnTagsString=a
      settings: SourceProductName=Simscape Electrical
  a : PMIOPort  Side=Right
  A : PMIOPort  Port=2  Side=Left
  connections:
  A/RConn1 -- 2/LConn1
  a/RConn1 -- 2/RConn1
  Ground83/LConn1 -- 2/LConn2 -- 2/LConn3
  Ground82/LConn1 -- 2/RConn2 -- 2/RConn3

== system IEEE123bus_v2019b_Phasor_DPL_ZIPload/46 Y PQ ==
  Controlled Current Source : powerlib/Electrical Sources/Controlled Current Source  Initialize=off  Source_Type=AC  Amplitude=0  Phase=0  Frequency=0  Measurements=None
      settings: SourceProductName=Simscape Electrical
  Embedded MATLAB Function : MATLAB Function  TreatAsAtomicUnit=on
  Gain4 : Gain  Gain=sqrt(2)
  Gain5 : Gain  Gain=1/sqrt(2)
  Memory1 : Memory
  Rc+jXc1 : powerlib/Elements/Series RLC Branch  LConnTagsString=__new0  RConnTagsString=__new0  BranchType=R  Resistance=1e6  Inductance=1.6 / (120*pi) * 2  SetiL0=off  InitialCurrent=0  Capacitance=1e-6  Setx0=off  InitialVoltage=0  Measurements=None
      settings: SourceProductName=Simscape Electrical
  Voltage Measurement1 : powerlib/Measurements/Voltage Measurement  PhasorSimulation=on  OutputType=Complex  PSBequivalent=0
      settings: SourceProductName=Simscape Electrical
  " 2" : PMIOPort  Tag=PMCPort  Side=Left
  " 3" : PMIOPort  Tag=PMCPort  Port=2  Side=Right
  wires:
  Embedded MATLAB Function/1(Iinj) -> Gain4/1
  Memory1/1 -> Controlled Current Source/1
  Gain5/1 -> Embedded MATLAB Function/1(Vmeas)
  Voltage Measurement1/1 -> [v]
  [v] -> Gain5/1
  Gain4/1 -> Memory1/1
  connections:
  Controlled Current Source/RConn1 -- Rc+jXc1/RConn1 -- Voltage Measurement1/LConn2 -- " 3"/RConn1
  Rc+jXc1/LConn1 -- " 2"/RConn1 -- Voltage Measurement1/LConn1 -- Controlled Current Source/LConn1

== system IEEE123bus_v2019b_Phasor_DPL_ZIPload/47 Y I ==
  Controlled Current Source : powerlib/Electrical Sources/Controlled Current Source  Initialize=off  Source_Type=AC  Amplitude=0  Phase=0  Frequency=0  Measurements=None
      settings: SourceProductName=Simscape Electrical
  Controlled Current Source1 : powerlib/Electrical Sources/Controlled Current Source  Initialize=off  Source_Type=AC  Amplitude=0  Phase=0  Frequency=0  Measurements=None
      settings: SourceProductName=Simscape Electrical
  Controlled Current Source2 : powerlib/Electrical Sources/Controlled Current Source  Initialize=off  Source_Type=AC  Amplitude=0  Phase=0  Frequency=0  Measurements=None
      settings: SourceProductName=Simscape Electrical
  Demux1 : Demux  Outputs=3
  Embedded MATLAB Function2 : MATLAB Function  TreatAsAtomicUnit=on
  Gain4 : Gain  Gain=sqrt(2)
  Gain5 : Gain  Gain=1/sqrt(2)
  Ground1 : powerlib/Elements/Ground  LConnTagsString=a
      settings: SourceProductName=Simscape Electrical
  Memory3 : Memory
  Mux5 : Mux  Inputs=3
  Rc+jXc1 : powerlib/Elements/Series RLC Branch  LConnTagsString=__new0  RConnTagsString=__new0  BranchType=R  Resistance=1e6  Inductance=1.6 / (120*pi) * 2  SetiL0=off  InitialCurrent=0  Capacitance=1e-6  Setx0=off  InitialVoltage=0  Measurements=None
      settings: SourceProductName=Simscape Electrical
  Rc+jXc2 : powerlib/Elements/Series RLC Branch  LConnTagsString=__new0  RConnTagsString=__new0  BranchType=R  Resistance=1e6  Inductance=1.6 / (120*pi) * 2  SetiL0=off  InitialCurrent=0  Capacitance=1e-6  Setx0=off  InitialVoltage=0  Measurements=None
      settings: SourceProductName=Simscape Electrical
  Rc+jXc3 : powerlib/Elements/Series RLC Branch  LConnTagsString=__new0  RConnTagsString=__new0  BranchType=R  Resistance=1e6  Inductance=1.6 / (120*pi) * 2  SetiL0=off  InitialCurrent=0  Capacitance=1e-6  Setx0=off  InitialVoltage=0  Measurements=None
      settings: SourceProductName=Simscape Electrical
  Voltage Measurement4 : powerlib/Measurements/Voltage Measurement  PhasorSimulation=on  OutputType=Complex  PSBequivalent=0
      settings: SourceProductName=Simscape Electrical
  Voltage Measurement5 : powerlib/Measurements/Voltage Measurement  PhasorSimulation=on  OutputType=Complex  PSBequivalent=0
      settings: SourceProductName=Simscape Electrical
  Voltage Measurement6 : powerlib/Measurements/Voltage Measurement  PhasorSimulation=on  OutputType=Complex  PSBequivalent=0
      settings: SourceProductName=Simscape Electrical
  " A" : PMIOPort  Tag=PMCPort  Side=Left
  " B" : PMIOPort  Tag=PMCPort  Port=2  Side=Left
  " C" : PMIOPort  Tag=PMCPort  Port=3  Side=Left
  wires:
  [vC] -> Mux5/3
  [vB] -> Mux5/2
  [vA] -> Mux5/1
  Gain5/1 -> Embedded MATLAB Function2/1(Vmeas)
  Mux5/1 -> Gain5/1
  Gain4/1 -> Memory3/1
  Embedded MATLAB Function2/1(Iinj) -> Gain4/1
  Demux1/3 -> Controlled Current Source2/1
  Voltage Measurement5/1 -> [vB]
  Voltage Measurement6/1 -> [vC]
  Demux1/1 -> Controlled Current Source/1
  Memory3/1 -> Demux1/1
  Demux1/2 -> Controlled Current Source1/1
  Voltage Measurement4/1 -> [vA]
  connections:
  Ground1/LConn1 -- Controlled Current Source/RConn1 -- Rc+jXc1/RConn1 -- Voltage Measurement4/LConn2 -- Controlled Current Source2/RConn1 -- Voltage Measurement6/LConn2 -- Rc+jXc3/RConn1 -- Voltage Measurement5/LConn2 -- Rc+jXc2/RConn1 -- Controlled Current Source1/RConn1
  Rc+jXc3/LConn1 -- Voltage Measurement6/LConn1 -- " C"/RConn1 -- Controlled Current Source2/LConn1
  Rc+jXc1/LConn1 -- Voltage Measurement4/LConn1 -- Controlled Current Source/LConn1 -- " A"/RConn1
  Controlled Current Source1/LConn1 -- Rc+jXc2/LConn1 -- Voltage Measurement5/LConn1 -- " B"/RConn1
